simulink model "sampleModel1665"  (R2023a)
settings: Solver=VariableStepAuto  StartTime=0.0  StopTime=10.0  RelTol=1e-3
libraries: hdlsllib x5, simulink x2
settings Model: Creator=user1  LastModifiedBy=user1

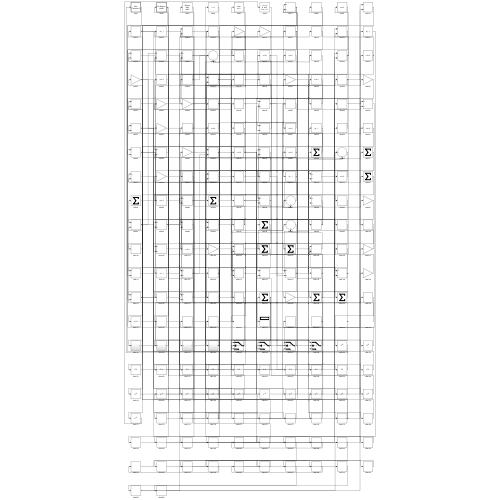
[thumbnail: Simulink's stored preview of the top-level diagram]
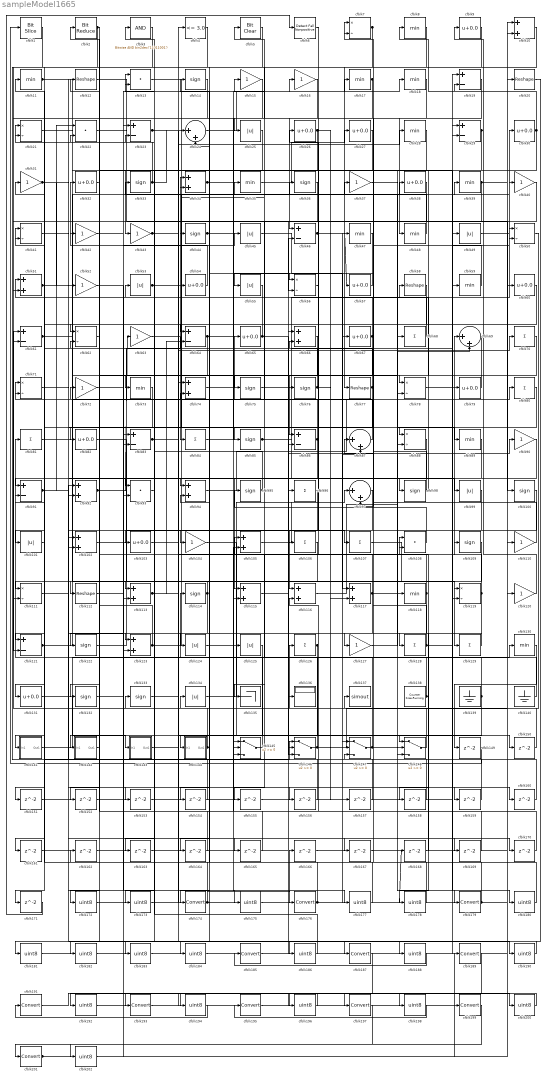
== system sampleModel1665 ==
  cfblk1 : hdlsllib/Logic and Bit Operations/Bit Slice  lidx=7  ridx=0
  cfblk{10,34,51,66,74,92,94,102,105,113,115..117,123} (14 alike) : Sum
  cfblk{14,33,36,44,75..76,85,95,98,100,109,114,122,132..133} (15 alike) : Signum
  cfblk{25,45,49,53,55,99,101,124..125,134} (10 alike) : Abs  SaturateOnIntegerOverflow=off
  cfblk{9,26..27,30,32,38,54,57,60,65,67,79,82,103,131} (15 alike) : Bias  Bias=0.0  SaturateOnIntegerOverflow=off
  cfblk{15..16,31,37,40,42..43,52,63,72,90,104,110,120,127} (15 alike) : Gain
  cfblk{68,70,80..81,84,96,106..107,126,128..129} (11 alike) : Sum  Inputs=+
  cfblk{13,22,93,108} (4 alike) : DotProduct  OutDataTypeStr=Inherit: Inherit via internal rule
  cfblk{8,11,17..18,28,35,39,47..48,59,73,89,118,130} (14 alike) : MinMax
  cfblk{7,21,41,50,56,62,71,78,88,111,119} (11 alike) : Product  Inputs=*/  RndMeth=Zero  SaturateOnIntegerOverflow=on
  cfblk{12,20,58,77,112} (5 alike) : Reshape
  cfblk{19,23,29,46,61,64,83,86,91,121} (10 alike) : Sum  Inputs=+-
  cfblk135 : Terminator
  cfblk136 : Display
  cfblk137 : ToWorkspace  VariableName=simout  SaveFormat=Timeseries  SampleTime=-1
  cfblk138 : hdlsllib/Sources/Counter Free-Running  NumBits=16  tsamp=-1
  cfblk139 : Ground
  cfblk140 : Ground
  cfblk141 : Subsystem
      settings: LibrarySourceBlock=|
      | hdlsllib/Ports &
      | Subsystems/Subsystem
  cfblk142 : Subsystem
      settings: LibrarySourceBlock=|
      | hdlsllib/Ports &
      | Subsystems/Subsystem
  cfblk143 : Subsystem
      settings: LibrarySourceBlock=|
      | hdlsllib/Ports &
      | Subsystems/Subsystem
  cfblk144 : Subsystem
      settings: LibrarySourceBlock=|
      | hdlsllib/Ports &
      | Subsystems/Subsystem
  cfblk{145..148} (4 alike) : Switch  SaturateOnIntegerOverflow=off  InputSameDT=off
  cfblk{149..171} (23 alike) : Delay  SampleTime=1
  cfblk{172..173,175,177..178,180..184,186,188,190,192,194,196,198,200,202} (19 alike) : DataTypeConversion  OutDataTypeStr=uint8  SaturateOnIntegerOverflow=off  RndMeth=Floor
  cfblk{174,176,179,185,187,189,191,193,195,197,199,201} (12 alike) : DataTypeConversion  SaturateOnIntegerOverflow=off  RndMeth=Floor
  cfblk2 : hdlsllib/Logic and Bit Operations/Bit Reduce  mode=AND
  cfblk{24,69,87,97} (4 alike) : Sum  Inputs=|++
  cfblk3 : simulink/Logic and Bit Operations/Bitwise Operator  logicop=AND  UseBitMask=on  BitMask=bin2dec('11011001')  BitMaskRealWorld=Stored Integer
      settings: LibrarySourceBlock=|
      | hdlsllib/Logic and Bit
      | Operations/Bitwise
      | Operator
  cfblk4 : hdlsllib/Logic and Bit Operations/Compare To Constant  relop=<=  const=3.0  OutDataTypeStr=boolean
  cfblk5 : simulink/Logic and Bit Operations/Bit Clear  iBit=0
      settings: LibrarySourceBlock=|
      | hdlsllib/Logic and Bit
      | Operations/Bit Clear
  cfblk6 : hdlsllib/Logic and Bit Operations/Detect Fall Nonpositive  vinit=0  OutDataTypeStr=boolean
  wires:
  cfblk121/1 -> cfblk35/1, cfblk177/1
  cfblk74/1 -> cfblk176/1
  cfblk122/1 -> cfblk65/1
  cfblk53/1 -> cfblk5/1, cfblk13/1
  cfblk79/1 -> cfblk75/1
  cfblk34/1 -> cfblk56/1, cfblk86/2
  cfblk124/1 -> cfblk97/1
  cfblk10/1 -> cfblk77/1
  cfblk141/1(Out1) -> cfblk130/1
  cfblk75/1 -> cfblk30/1
  cfblk1/1 -> cfblk146/1
  cfblk119/1 -> cfblk69/1, cfblk158/1
  cfblk67/1 -> cfblk51/1, cfblk83/2
  cfblk49/1 -> cfblk50/1
  cfblk23/1 -> cfblk85/1, cfblk159/1
  cfblk61/1 -> cfblk98/1, cfblk87/2
  cfblk134/1 -> cfblk108/1
  cfblk92/1 -> cfblk63/1, cfblk107/1
  cfblk138/1 -> cfblk3/1, cfblk178/1
  cfblk114/1 -> cfblk111/1, cfblk182/1
  cfblk87/1 -> cfblk15/1
  cfblk11/1 -> cfblk113/1, cfblk99/1
  cfblk102/1 -> cfblk34/1
  cfblk54/1 -> cfblk32/1
  cfblk62/1 -> cfblk12/1
  cfblk31/1 -> cfblk52/1, cfblk167/1
  cfblk76/1 -> cfblk41/1, cfblk117/2
  cfblk51/1 -> cfblk88/1, cfblk153/1
  cfblk123/1 -> cfblk40/1, cfblk22/2
  cfblk82/1 -> cfblk129/1
  cfblk131/1 -> cfblk143/1(In1)
  cfblk140/1 -> cfblk114/1
  cfblk94/1 -> cfblk49/1
  cfblk16/1 -> cfblk46/1
  cfblk86/1 -> cfblk123/1, cfblk71/2
  cfblk13/1 -> cfblk79/1
  cfblk98/1 -> cfblk58/1, cfblk66/2
  cfblk36/1 -> cfblk56/2
  cfblk19/1 -> cfblk48/1
  cfblk110/1 -> cfblk72/1
  cfblk120/1 -> cfblk19/2
  cfblk63/1 -> cfblk84/1
  cfblk25/1 -> cfblk43/1
  cfblk104/1 -> cfblk148/1
  cfblk21/1 -> cfblk125/1
  cfblk47/1 -> cfblk104/1
  cfblk71/1 -> cfblk123/2
  cfblk73/1 -> cfblk92/2
  cfblk81/1 -> cfblk59/1
  cfblk28/1 -> cfblk144/1(In1)
  cfblk64/1 -> cfblk73/1, cfblk76/1
  cfblk118/1 -> cfblk124/1, cfblk36/1
  cfblk85/1 -> cfblk50/2, cfblk119/2
  cfblk126/1 -> cfblk145/3, cfblk152/1
  cfblk116/1 -> cfblk68/1
  cfblk50/1 -> cfblk137/1
  cfblk112/1 -> cfblk44/1
  cfblk26/1 -> cfblk132/1, cfblk157/1
  cfblk56/1 -> cfblk26/1
  cfblk91/1 -> cfblk22/1, cfblk165/1
  cfblk83/1 -> cfblk45/1, cfblk169/1
  cfblk42/1 -> cfblk17/1
  cfblk32/1 -> cfblk112/1
  cfblk70/1 -> cfblk103/1
  cfblk80/1 -> cfblk148/2
  cfblk101/1 -> cfblk41/2
  cfblk66/1 -> cfblk122/1
  cfblk88/1 -> cfblk115/1
  cfblk24/1 -> cfblk18/1
  cfblk60/1 -> cfblk174/1
  cfblk12/1 -> cfblk100/1
  cfblk145/1 -> cfblk81/1
  cfblk43/1 -> cfblk28/1, cfblk38/1
  cfblk143/1(Out1) -> cfblk109/1
  cfblk77/1 -> cfblk54/1, cfblk121/1
  cfblk35/1 -> cfblk27/1
  cfblk48/1 -> cfblk33/1
  cfblk90/1 -> cfblk94/1
  cfblk3/1 -> cfblk101/1
  cfblk45/1 -> cfblk117/1
  cfblk144/1(Out1) -> cfblk134/1, cfblk34/2
  cfblk59/1 -> cfblk7/1
  cfblk39/1 -> cfblk10/1, cfblk121/2
  cfblk57/1 -> cfblk55/1
  cfblk146/1 -> cfblk120/1, cfblk14/1
  cfblk58/1 -> cfblk141/1(In1)
  cfblk18/1 -> cfblk97/2
  cfblk113/1 -> cfblk70/1, cfblk64/2
  cfblk14/1 -> cfblk51/2
  cfblk2/1 -> cfblk61/2, cfblk82/1
  cfblk129/1 -> cfblk128/1
  cfblk127/1 -> cfblk39/1
  cfblk125/1 -> cfblk142/1(In1)
  cfblk41/1 -> cfblk102/1
  cfblk9/1 -> cfblk131/1
  cfblk37/1 -> cfblk179/1
  cfblk38/1 -> cfblk135/1
  cfblk100/1 -> cfblk116/1
  cfblk117/1 -> cfblk42/1, cfblk69/2, cfblk127/1
  cfblk17/1 -> cfblk115/2, cfblk111/2
  cfblk15/1 -> cfblk64/1
  cfblk142/1(Out1) -> cfblk2/1
  cfblk128/1 -> cfblk87/1, cfblk80/1
  cfblk7/1 -> cfblk25/1, cfblk24/2
  cfblk115/1 -> cfblk90/1
  cfblk44/1 -> cfblk89/1, cfblk78/2
  cfblk33/1 -> cfblk21/1, cfblk24/1
  cfblk22/1 -> cfblk118/1
  cfblk46/1 -> cfblk57/1, cfblk147/2
  cfblk84/1 -> cfblk16/1
  cfblk148/1 -> cfblk126/1
  cfblk69/1 -> cfblk86/1
  cfblk105/1 -> cfblk47/1
  cfblk30/1 -> cfblk8/1, cfblk78/1
  cfblk108/1 -> cfblk95/1
  cfblk6/1 -> cfblk106/1
  cfblk65/1 -> cfblk136/1, cfblk62/1, cfblk148/3
  cfblk29/1 -> cfblk88/2, cfblk9/1
  cfblk139/1 -> cfblk71/1, cfblk146/3
  cfblk95/1 -> cfblk93/1, cfblk13/2
  cfblk107/1 -> cfblk119/1
  cfblk147/1 -> cfblk105/1, cfblk170/1
  cfblk8/1 -> cfblk91/1
  cfblk68/1 -> cfblk11/1
  cfblk99/1 -> cfblk102/2
  cfblk130/1 -> cfblk149/1
  cfblk149/1 -> cfblk1/1
  cfblk103/1 -> cfblk150/1
  cfblk150/1 -> cfblk61/1
  cfblk55/1 -> cfblk151/1
  cfblk151/1 -> cfblk19/1
  cfblk152/1 -> cfblk113/2
  cfblk153/1 -> cfblk105/2
  cfblk109/1 -> cfblk154/1
  cfblk154/1 -> cfblk21/2
  cfblk97/1 -> cfblk155/1
  cfblk155/1 -> cfblk147/1
  cfblk132/1 -> cfblk156/1
  cfblk156/1 -> cfblk146/2
  cfblk157/1 -> cfblk23/2
  cfblk158/1 -> cfblk145/2
  cfblk159/1 -> cfblk147/3
  cfblk72/1 -> cfblk160/1
  cfblk160/1 -> cfblk92/1
  cfblk89/1 -> cfblk161/1
  cfblk161/1 -> cfblk66/1
  cfblk162/1 -> cfblk93/2
  cfblk27/1 -> cfblk163/1
  cfblk163/1 -> cfblk46/2
  cfblk5/1 -> cfblk164/1
  cfblk164/1 -> cfblk83/1
  cfblk165/1 -> cfblk145/1
  cfblk166/1 -> cfblk10/2
  cfblk167/1 -> cfblk7/2
  cfblk168/1 -> cfblk108/2
  cfblk169/1 -> cfblk116/2
  cfblk170/1 -> cfblk62/2
  cfblk106/1 -> cfblk171/1
  cfblk171/1 -> cfblk6/1
  cfblk4/1 -> cfblk172/1
  cfblk172/1 -> cfblk67/1
  cfblk93/1 -> cfblk173/1
  cfblk173/1 -> cfblk4/1
  cfblk174/1 -> cfblk166/1, cfblk91/2, cfblk53/1
  cfblk52/1 -> cfblk175/1
  cfblk175/1 -> cfblk60/1
  cfblk176/1 -> cfblk168/1, cfblk31/1
  cfblk177/1 -> cfblk74/1
  cfblk178/1 -> cfblk74/2
  cfblk179/1 -> cfblk162/1, cfblk94/2
  cfblk78/1 -> cfblk180/1
  cfblk180/1 -> cfblk37/1
  cfblk20/1 -> cfblk181/1
  cfblk181/1 -> cfblk29/2
  cfblk182/1 -> cfblk20/1
  cfblk96/1 -> cfblk183/1
  cfblk183/1 -> cfblk29/1
  cfblk40/1 -> cfblk184/1
  cfblk184/1 -> cfblk96/1
  cfblk111/1 -> cfblk186/1
  cfblk186/1 -> cfblk133/1
  cfblk133/1 -> cfblk188/1
  cfblk188/1 -> cfblk185/1
  cfblk185/1 -> cfblk190/1
  cfblk190/1 -> cfblk187/1
  cfblk187/1 -> cfblk192/1
  cfblk192/1 -> cfblk189/1
  cfblk189/1 -> cfblk194/1
  cfblk194/1 -> cfblk191/1
  cfblk191/1 -> cfblk196/1
  cfblk196/1 -> cfblk193/1
  cfblk193/1 -> cfblk198/1
  cfblk198/1 -> cfblk195/1
  cfblk199/1 -> cfblk201/1
  cfblk195/1 -> cfblk200/1
  cfblk200/1 -> cfblk197/1
  cfblk201/1 -> cfblk110/1, cfblk23/1
  cfblk197/1 -> cfblk202/1
  cfblk202/1 -> cfblk199/1

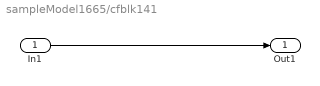
== system sampleModel1665/cfblk141 ==
  In1 : Inport
  Out1 : Outport
  wires:
  In1/1 -> Out1/1

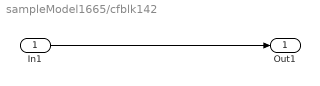
== system sampleModel1665/cfblk142 ==
  In1 : Inport
  Out1 : Outport
  wires:
  In1/1 -> Out1/1

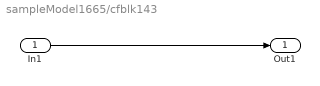
== system sampleModel1665/cfblk143 ==
  In1 : Inport
  Out1 : Outport
  wires:
  In1/1 -> Out1/1

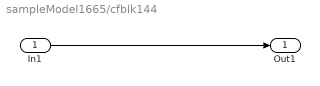
== system sampleModel1665/cfblk144 ==
  In1 : Inport
  Out1 : Outport
  wires:
  In1/1 -> Out1/1
